simulink model "Aplicacion7"  (R2022b)
settings: Solver=ode45  StartTime=0.0  StopTime=30  RelTol=1e-3  AbsTol=1e-6
undefined symbols (not defined in the file): sfunxy2
libraries: neural x1
settings Model: TunableVars=prueba  TunableVarsStorageClass=Auto  Creator=matthew  LastModifiedBy=PC-LUISMIGUEL
settings SolverCC: AutoScaleAbsTol=off
settings DataIOCC: SaveFormat=Array  SignalLoggingSaveFormat=ModelDataLogs  SaveOutput=off  ReturnWorkspaceOutputs=off  SignalLoggingName=sigsOut
settings OptimizationCC: BooleanDataType=off  InitFltsAndDblsToZero=on  LifeSpan=inf
settings DebuggingCC: SaveWithParameterizedLinksMsg=none  UnderspecifiedInitializationDetection=Classic  MergeDetectMultiDrivingBlocksExec=none  SignalResolutionControl=TryResolveAllWithWarning  MultiTaskDSMMsg=warning  MultiTaskCondExecSysMsg=none  UnconnectedInputMsg=warning  UnconnectedOutputMsg=warning  UnconnectedLineMsg=warning  SFUnexpectedBacktrackingDiag=warning  SFNoUnconditionalDefaultTransitionDiag=warning  SFExecutionAtInitializationDiag=none  SFMachineParentedDataDiag=warning  ArithmeticOperatorsInVariantConditions=warning
settings HardwareCC: ProdBitPerPointer=32  ProdBitPerSizeT=32  ProdBitPerPtrDiffT=32  ProdLargestAtomicFloat=None  ProdIntDivRoundTo=Undefined  ProdEndianess=Unspecified  ProdWordSize=32  ProdHWDeviceType=32-bit Generic  TargetUnknown=on
settings ModelReferenceCC: PropagateSignalLabelsOutOfModel=off
settings RTWCC: TemplateMakefile=grt_vc.tmf
settings CodeAppCC: StateflowObjectComments=on
settings GRTTargetCC: TargetFcnLib=ansi_tfl_tmw.mat  TargetLangStandard=C89/C90 (ANSI)  CombineOutputUpdateFcns=off  GRTInterface=on
settings ConfigComp: CovMetricSettings=dw  CovSaveCumulativeToWorkspaceVar=on  CovSaveSingleToWorkspaceVar=on

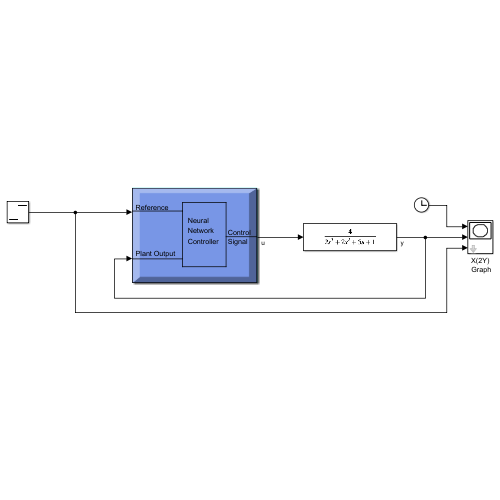
[thumbnail: Simulink's stored preview of the top-level diagram]
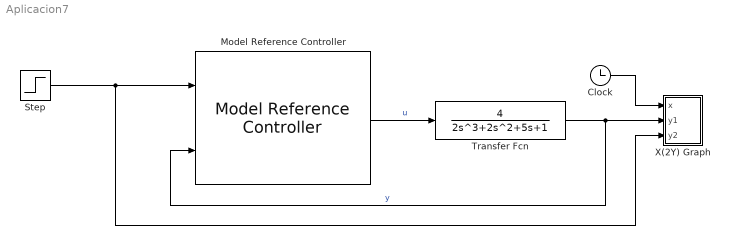
== system Aplicacion7 ==
  Clock : Clock
  Model Reference Controller : neural/Control Systems/Model Reference Controller  Nrc=2  Nic=2  Njc=2  IW_y=[0.77641519056418795142 -0.16577513390090925505;0.012578940199918451845 0.94806458766607792921;-0.57689810704896071769 -0.87231832403340392457;-0.5519008314371808277 -0.17098069188326880941;0.37822288177970575518 -1.0847242617705978862]  IW_u=[0.78315480105239487774 0.58759704951376956483;-0.65773234832888149981 0.10658518116996548719;-0.82184272402423685921 0.58361193960069990272;-1.1561290364423346677 0.68133434017005967132;0.92883582626422545037 0.50241910858360105951]  IW_r=[-0.92844427937509255155 0.84202224475965625761;0.15702837835753963303 1.3924025620798987646;1.055942104553624139 -0.73944497521498575576;0.206116860472833896 -0.97249466062772249586;0.92371473801467218756 -0.17146573314229981988]  B1_c=[-1.6924672550803208093;-0.94688328590505599358;0.18770465037941333475;-0.93857255665581473814;1.8686694752805750319]  B2_c=-0.20906232937548691053  LW_c=[-0.83483594116733150781 0.34488531369837405194 1.0784415791270933749 -0.23218114464295022681 0.14647509556240786988]  retraining_c=2  max_i_int=10  min_i_int=6  max_r_int=8  min_r_int=4  Ts=0.1  S1=5  Ni=2  Nj=2  sim_file=ModeloPlanta7  trainfun=trainlm  Use_validation=0  Use_Testing=0  Use_Inc_training=0  Use_previous_weights=1  max_i=0.5  min_i=0  max_r=1  min_r=0  sam_training=800  sam_training_c=300  epochs=300  epochs_c=650  minp=0.0078223463482635091637  maxp=0.43193411146680532608  mint=0  maxt=0.43193411146680532608  Normalize=0  IW=[1.70282097286769174 2.1126047664248797098;0.00093606485748506538993 0.00082568390645187635709;1.4937351723960541339 3.8938386580219219724;0.63812927834029409269 2.6328520891207256582;-0.018186916131577253453 -0.02488164794055726381]  LW1_2=[4.119913068524532207 3.6603584682804428674;-0.13436245172639749157 0.064726704987180416762;-0.84025004492917054755 -4.2823334795164544886;3.7413083189245681659 3.3850630462326756209;-0.46965566191949592589 0.22642853201464577251]  LW2_1=[-0.0038649816285129322095 -19.094434783722672222 0.0029335480787683579536 2.1407732057304489359 -3.8007218871128869431]  B1=[-0.37527071907761516689;0.73016772477094160632;5.1350474368513596701;3.2215686432577710363;-1.4301758090511782484]  B2=6.3689870568413073926  S1c=5  Limit_output=0  min_output=-Inf  max_output=Inf  Ref_file=ModeloPlantaReferencia7
  Step : Step  Time=0  SampleTime=0
  Transfer Fcn : TransferFcn  Numerator=[4]  Denominator=[2 2 5 1]
  X(2Y) Graph : Subsystem  LoadFcn=sfunxy2([],[],[],'LoadBlock')  StartFcn=sfunxy2([],[],[],'Start')  StopFcn=sfunxy2([],[],[],'Stop')  mask(X(2Y) scope.){xmin=0, xmax=30, ymin=0, ymax=1.5, st=-1}
      mask prompts: xmin "x-min:"; xmax "x-max:"; ymin "y-min:"; ymax "y-max:"; st "Sample time:"
      mask help: X(2Y) scope using MATLAB graph window. First input is used as time base. Enter plotting ranges.
      settings: CopyFcn=sfunxy2([],[],[],'CopyBlock')  DeleteFcn=sfunxy2([],[],[],'DeleteBlock')  NameChangeFcn=sfunxy2([],[],[],'NameChange')
      mask Help: This block can be used to explore limit cycles. Look at the m-file sfunxy.m to see how it works.
      mask Display: plot([.05 .95 .95 .05 .05],[.45 .45 .95 .95 .45], 0.5+cos(0:0.1:2*pi)*0.3,0.7+sin(0:0.1:2*pi)*0.2)
  wires:
  Transfer Fcn/1 -> X(2Y) Graph/2(y1), Model Reference Controller/2  "y"
  Model Reference Controller/1 -> Transfer Fcn/1  "u"
  Clock/1 -> X(2Y) Graph/1(x)
  Step/1 -> X(2Y) Graph/3(y2), Model Reference Controller/1

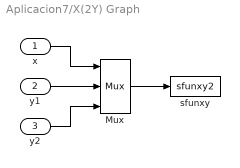
== system Aplicacion7/X(2Y) Graph ==
  x : Inport
  y1 : Inport  Port=2
  y2 : Inport  Port=3
  Mux : Mux  Inputs=3
  sfunxy : S-Function  FunctionName=sfunxy2  Parameters=[xmin xmax ymin ymax], st  SFunctionDeploymentMode=off  EnableBusSupport=off
  wires:
  y2/1 -> Mux/3
  y1/1 -> Mux/2
  x/1 -> Mux/1
  Mux/1 -> sfunxy/1
